simulink model "bh_explained_force_sensor"  (R2018a)
settings: Solver=ode15s  StartTime=0.0  StopTime=20  MaxStep=0.01  RelTol=1e-3  EnableMultiTasking=on
model workspace (MAT data in the model file):
  c = 1.2
  k = 9
  m = 1
libraries: fl_lib x11, nesl_utility x7
Description:
  | Copyright 2014 The MathWorks, Inc.
settings Model: Creator=smiller  LastModifiedBy=bhorton
settings DataIOCC: LimitDataPoints=on  SaveFormat=Array
settings OptimizationCC: LifeSpan=inf
settings DebuggingCC: UnderspecifiedInitializationDetection=Classic  MergeDetectMultiDrivingBlocksExec=none  SolverPrmCheckMsg=warning  AllowSymbolicDim=off  StateNameClashWarn=warning  SFUnexpectedBacktrackingDiag=warning  SFNoUnconditionalDefaultTransitionDiag=warning  SFExecutionAtInitializationDiag=none
settings HardwareCC: ProdBitPerPointer=32  ProdBitPerSizeT=32  ProdBitPerPtrDiffT=32  ProdLargestAtomicFloat=None  ProdIntDivRoundTo=Undefined  ProdEndianess=Unspecified  ProdWordSize=32  ProdHWDeviceType=32-bit Generic
settings ModelReferenceCC: PropagateSignalLabelsOutOfModel=off
settings CodeAppCC: StateflowObjectComments=on
settings GRTTargetCC: TargetLangStandard=C89/C90 (ANSI)  GeneratePreprocessorConditionals=Disable all
settings ConfigComp: CovMetricSettings=dw  CovHtmlReporting=on  CovSaveCumulativeToWorkspaceVar=on  CovSaveSingleToWorkspaceVar=on  CovExternalEMLEnable=off  CovSFcnEnable=off
settings SimscapeCC: SimscapeNormalizeSystem=off

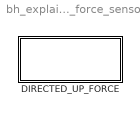
== system bh_explained_force_sensor ==
  DIRECTED_UP_FORCE : Subsystem

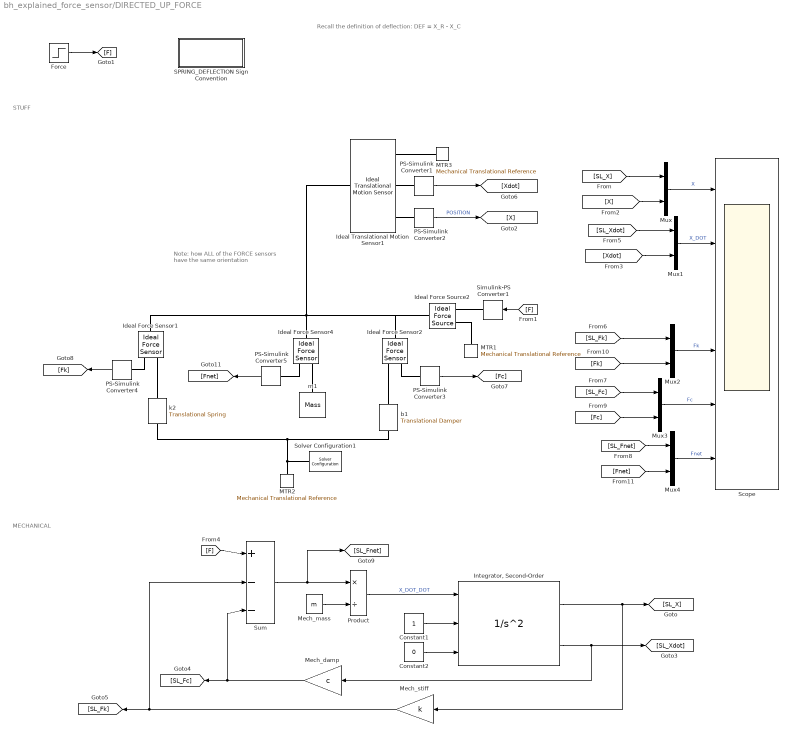
== system bh_explained_force_sensor/DIRECTED_UP_FORCE ==
  note: Note: how ALL of the FORCE sensors
      | have the same orientation
  note: STUFF
  note: Recall the definition of deflection:
      |
      |          DEF = X_R - X_C
  note: MECHANICAL
  Constant1 : Constant
  Constant2 : Constant  Value=0
  Force : Step  Time=15  After=9  SampleTime=0
      settings: AttributesFormatString=|
      | Time of step = %<Time>
      | Final value = %<After>
  Ideal Force Sensor1 : fl_lib/Mechanical/Mechanical Sensors/Ideal Force Sensor
  Ideal Force Sensor2 : fl_lib/Mechanical/Mechanical Sensors/Ideal Force Sensor
  Ideal Force Sensor4 : fl_lib/Mechanical/Mechanical Sensors/Ideal Force Sensor
  Ideal Force Source2 : fl_lib/Mechanical/Mechanical Sources/Ideal Force Source
  Ideal Translational Motion Sensor1 : fl_lib/Mechanical/Mechanical Sensors/Ideal Translational Motion Sensor  offset=1 m
      settings: AttributesFormatString=INITIAL_POS= %<offset>
  "Integrator, Second-Order" : SecondOrderIntegrator  ICSourceX=external  UpperLimitX=Mech.x_max  LowerLimitX=Mech.x_min  ICSourceDXDT=external  ReinitDXDTwhenXreachesSaturation=on
  MTR1 : fl_lib/Mechanical/Translational Elements/Mechanical Translational Reference
  MTR2 : fl_lib/Mechanical/Translational Elements/Mechanical Translational Reference
  MTR3 : fl_lib/Mechanical/Translational Elements/Mechanical Translational Reference
  Mech_damp : Gain  Gain=c
  Mech_mass : Constant  Value=m
  Mech_stiff : Gain  Gain=k
  Mux{,1..4} (5 alike) : Mux  Inputs=2
  PS-Simulink Converter1 : nesl_utility/PS-Simulink Converter  PhysicalDomain=network_engine_domain  SubClassName=ps_output  LeftPortType=input  RightPortType=output  PseudoPeriodic=off  Frequencies=[]  Unit=m/s  AffineConversion=off
  PS-Simulink Converter2 : nesl_utility/PS-Simulink Converter  PhysicalDomain=network_engine_domain  SubClassName=ps_output  LeftPortType=input  RightPortType=output  PseudoPeriodic=off  Frequencies=[]  Unit=m  AffineConversion=off
  PS-Simulink Converter3 : nesl_utility/PS-Simulink Converter  PhysicalDomain=network_engine_domain  SubClassName=ps_output  LeftPortType=input  RightPortType=output  PseudoPeriodic=off  Frequencies=[]  Unit=N  AffineConversion=off
  PS-Simulink Converter4 : nesl_utility/PS-Simulink Converter  PhysicalDomain=network_engine_domain  SubClassName=ps_output  LeftPortType=input  RightPortType=output  PseudoPeriodic=off  Frequencies=[]  Unit=N  AffineConversion=off
  PS-Simulink Converter5 : nesl_utility/PS-Simulink Converter  PhysicalDomain=network_engine_domain  SubClassName=ps_output  LeftPortType=input  RightPortType=output  PseudoPeriodic=off  Frequencies=[]  Unit=N  AffineConversion=off
  Product : Product  Inputs=*/
  SPRING_DEFLECTION Sign Convention : Subsystem
  Scope : Scope  NumInputPorts=6
  Simulink-PS Converter1 : nesl_utility/Simulink-PS Converter  PhysicalDomain=network_engine_domain  SubClassName=ps_input  LeftPortType=input  RightPortType=output  PseudoPeriodic=off  Frequencies=[]  NoiseDistribution=none  NoiseParameters=[]  Unit=N  AffineConversion=off  FilteringAndDerivatives=zero  SimscapeFilterOrder=1  InputFilterTimeConstant=.001  UdotUserProvided=0
  Solver Configuration1 : nesl_utility/Solver Configuration  PhysicalDomain=network_engine_domain  SubClassName=solver  LeftPortType=input  RightPortType=generic  Tones=[]  Harmonics=[]  SimulateNoise=off  Profile=off  UseLocalSampling=off  EnableSwitchedLinearOptims=on  FrequencyDomain=off  UseCCode=off  RelTol=0.001  AbsTol=1e-06  MinStep=1e-09  ToWorkspace=off  RevertToSquareIcSolve=off  NumHomotopyIterations=100  PhasorMode=off  PhasorModeNumHarmonics=1  DoDC=off  ResidualTolerance=1e-9  UseLocalSolver=off  LocalSolverChoice=NE_BACKWARD_EULER_ADVANCER  LocalSolverSampleTime=.001  DoFixedCost=off  MaxNonlinIter=12  MaxModeIter=2  LinearAlgebra=Sparse  EquationFormulation=NE_TIME_EF  DelaysMemoryBudget=1024  AutomaticFiltering=on  FilteringTimeConstant=0.001
  Sum : Sum  Inputs=+|-|-
  b1 : fl_lib/Mechanical/Translational Elements/Translational Damper  D=c N/(m/s)  v_specify=off  v_priority=None  v=0 m/s  v_nominal_specify=off  v_nominal_unit=m/s  v_nominal_value=1  f_specify=off  f_priority=None  f=0 N  f_nominal_specify=off  f_nominal_unit=N  f_nominal_value=1
  k2 : fl_lib/Mechanical/Translational Elements/Translational Spring  spr_rate=k N/m  v_specify=off  v_priority=None  v=0 m/s  v_nominal_specify=off  v_nominal_unit=m/s  v_nominal_value=1  f_specify=off  f_priority=None  f=0 N  f_nominal_specify=off  f_nominal_unit=N  f_nominal_value=1  x_specify=on  x_priority=High  x=1 m  x_nominal_specify=off  x_nominal_unit=m  x_nominal_value=1
      settings: AttributesFormatString=DEF_X = %<x>
  m1 : fl_lib/Mechanical/Translational Elements/Mass  mass=m kg  v_specify=on  v_priority=None  v=0 m/s  v_nominal_specify=off  v_nominal_unit=m/s  v_nominal_value=1  f_specify=off  f_priority=None  f=0 N  f_nominal_specify=off  f_nominal_unit=N  f_nominal_value=1
      settings: AttributesFormatString=V0 = %<v>
  wires:
  Force/1 -> [F]
  PS-Simulink Converter2/1 -> [X]  "POSITION"
  "Integrator, Second-Order"/2 -> Mech_damp/1, [SL_Xdot]
  Mech_damp/1 -> [SL_Fc], Sum/3
  Constant1/1 -> "Integrator, Second-Order"/2
  "Integrator, Second-Order"/1 -> Mech_stiff/1, [SL_X]
  Constant2/1 -> "Integrator, Second-Order"/3
  Mech_stiff/1 -> [SL_Fk], Sum/2
  Product/1 -> "Integrator, Second-Order"/1  "X_DOT_DOT"
  Mech_mass/1 -> Product/2
  Sum/1 -> [SL_Fnet], Product/1
  [F] -> Sum/1
  PS-Simulink Converter1/1 -> [Xdot]
  PS-Simulink Converter3/1 -> [Fc]
  PS-Simulink Converter4/1 -> [Fk]
  [SL_X] -> Mux/1
  [X] -> Mux/2
  [SL_Xdot] -> Mux1/1
  [Xdot] -> Mux1/2
  [SL_Fc] -> Mux3/1
  [SL_Fk] -> Mux2/1
  [Fnet] -> Mux4/2
  [Fc] -> Mux3/2
  [Fk] -> Mux2/2
  Mux4/1 -> Scope/6  "Fnet"
  Mux3/1 -> Scope/5  "Fc"
  Mux2/1 -> Scope/4  "Fk"
  Mux/1 -> Scope/1  "X"
  Mux1/1 -> Scope/2  "X_DOT"
  [F] -> Simulink-PS Converter1/1
  [SL_Fnet] -> Mux4/1
  PS-Simulink Converter5/1 -> [Fnet]
  connections:
  Ideal Translational Motion Sensor1/RConn3 -- PS-Simulink Converter2/LConn1
  MTR3/LConn1 -- Ideal Translational Motion Sensor1/RConn1
  MTR2/LConn1 -- b1/RConn1 -- k2/RConn1 -- Solver Configuration1/RConn1
  Ideal Force Sensor1/LConn1 -- Ideal Translational Motion Sensor1/LConn1 -- Ideal Force Sensor2/LConn1 -- Ideal Force Source2/LConn1 -- Ideal Force Sensor4/LConn1
  Ideal Force Sensor1/RConn1 -- k2/LConn1
  Ideal Translational Motion Sensor1/RConn2 -- PS-Simulink Converter1/LConn1
  PS-Simulink Converter4/LConn1 -- Ideal Force Sensor1/RConn2
  Simulink-PS Converter1/RConn1 -- Ideal Force Source2/RConn1
  Ideal Force Source2/RConn2 -- MTR1/LConn1
  Ideal Force Sensor2/RConn1 -- b1/LConn1
  PS-Simulink Converter3/LConn1 -- Ideal Force Sensor2/RConn2
  m1/LConn1 -- Ideal Force Sensor4/RConn1
  PS-Simulink Converter5/LConn1 -- Ideal Force Sensor4/RConn2

== system bh_explained_force_sensor/DIRECTED_UP_FORCE/SPRING_DEFLECTION Sign Convention ==
  note: Recall the definition of deflection:
      |
      |          DEF = X_R - X_C
  note: deflection is NEGATIVE (-)
  note: deflection is POSITIVE (+)
